simulink model "CACC_system_struct"  (Simulink 8.2)
settings: Solver=ode1  SolverMode=SingleTasking  StartTime=0.0  StopTime=inf  FixedStep=0.01  RelTol=1e-3
PreLoadFcn:
  | numd_dvsp = [0.3579 0 -0.3579];
  | dend_dvsp = [1 -1.846 0.8535];
  | simpleacc_param
PostLoadFcn:
  | , if any(exist('dsrtsu_mdlpostloadfcn', 'file') == [2, 3, 6]), try dsrtsu_mdlpostloadfcn('Execute', bdroot); catch fprintf('Error in PostLoadFcn (dsrtsu_mdlpostloadfcn) for model "%s":\n %s\n', bdroot, lasterr); end, end,
undefined symbols (not defined in the file or in its folder): command_mode, max_accel_m_s2, override_enabled, speed_command_m_s, wrench_effort_command
libraries: carma_platform x3, dsrc_transmitter x2, rtitttasklib x2, lightbar x2, srx_platform x1
(part 4 of 4)

== matlab function CACC Control Code 1/Coordination/MATLAB Function ==
  data: u input double; y output double
function y = fcn(u)
%#codegen

y=veh_pos(u);


function y_out=veh_pos(x)

%N=length(x);
cacc_grp_len=x(16);

z=zeros(1,15);
        if (cacc_grp_len == 2)                %% always put the subject vehicle at Virtual Position 1 in the Vector Forming            
                A=[x(2); x(5)];
                b=[x(3); x(6)];            
        elseif (cacc_grp_len == 3)            
                A=[x(2); x(5); x(8)];
                b=[x(3); x(6); x(9)];             
        elseif (cacc_grp_len == 4)           
                A=[x(2); x(5); x(8); x(11)];
                b=[x(3); x(6); x(9); x(12)];          
        elseif (cacc_grp_len == 5)            
                A=[x(2); x(5); x(8); x(11); x(14)];
                b=[x(3); x(6); x(9); x(12); x(15)];            
        else
             A=[x(2)];
             b=[x(3)];
        end
    
    a=A\b;
 
    alpha=atan(a(1));    %% angle of moving axle w.r.t. to East of the original coordinate system
    
    alpha=pi/2.0-alpha;  %% angle of moving axle w.r.t. to North of the original coordinate system
    alpha=-alpha;        %% so that the original y-axis is in the Miving Axle direction;
    
    
    if (cacc_grp_len == 2)                %% always put the subject vehicle at Virtual Position 1 in the Vector Forming         
            p1_2=Coord_Trans(alpha,A(1),b(1),A(2),b(2));
            tmp=[0 p1_2(2)];
            [Ord, Ind]=sort(tmp, 'descend');
            
            z(1)=x(1); %%BSM1: ID
            z(2)=Ind(1); %%BSM1: Contol Pos
            z(3)=0; %%BSM1: Lane ID
            z(4)=x(4); %%BSM2: ID
            z(5)=Ind(2); %%BSM2: Contol Pos
            z(6)=0; %%BSM2: Lane ID
            z(7)=-1; %%BSM3: ID
            z(8)=-1; %%BSM3: Contol Pos
            z(9)=-1; %%BSM3: Lane ID
            z(10)=-1; %%BSM4: ID
            z(11)=-1; %%BSM4: Contol Pos
            z(12)=-1; %%BSM4: Lane ID
            z(13)=-1; %%BSM5: ID
            z(14)=-1; %%BSM5: Contol Pos
            z(15)=-1; %%BSM5: Lane ID

            
   elseif (cacc_grp_len == 3)
            p1_2=Coord_Trans(alpha,A(1),b(1),A(2),b(2));
            p1_3=Coord_Trans(alpha,A(1),b(1),A(3),b(3));
            tmp=[0 p1_2(2) p1_3(2)];
            [Ord, Ind]=sort(tmp, 'descend');
            
            z(1)=x(1); %%BSM1: ID
            z(2)=Ind(1); %%BSM1: Contol Pos
            z(3)=0; %%BSM1: Lane ID
            z(4)=x(4); %%BSM2: ID
            z(5)=Ind(2); %%BSM2: Contol Pos
            z(6)=0; %%BSM2: Lane ID
            z(7)=x(7); %%BSM3: ID
            z(8)=Ind(3); %%BSM3: Contol Pos
            z(9)=0; %%BSM3: Lane ID
            z(10)=-1; %%BSM4: ID
            z(11)=-1; %%BSM4: Contol Pos
            z(12)=-1; %%BSM4: Lane ID
            z(13)=-1; %%BSM5: ID
            z(14)=-1; %%BSM5: Contol Pos
            z(15)=-1; %%BSM5: Lane ID
                     
    elseif (cacc_grp_len == 4)
            p1_2=Coord_Trans(alpha,A(1),b(1),A(2),b(2));
            p1_3=Coord_Trans(alpha,A(1),b(1),A(3),b(3));
            p1_4=Coord_Trans(alpha,A(1),b(1),A(4),b(4));
            tmp=[0 p1_2(2) p1_3(2) p1_4(2)];
            [Ord, Ind]=sort(tmp, 'descend');
            
            z(1)=x(1); %%BSM1: ID
            z(2)=Ind(1); %%BSM1: Contol Pos
            z(3)=0; %%BSM1: Lane ID
            z(4)=x(4); %%BSM2: ID
            z(5)=Ind(2); %%BSM2: Contol Pos
            z(6)=0; %%BSM2: Lane ID
            z(7)=x(7); %%BSM3: ID
            z(8)=Ind(3); %%BSM3: Contol Pos
            z(9)=0; %%BSM3: Lane ID
            z(10)=x(10); %%BSM4: ID
            z(11)=Ind(4); %%BSM4: Contol Pos
            z(12)=0; %%BSM4: Lane ID
            z(13)=-1; %%BSM5: ID
            z(14)=-1; %%BSM5: Contol Pos
            z(15)=-1; %%BSM5: Lane ID
                
    elseif (cacc_grp_len == 5)
            p1_2=Coord_Trans(alpha,A(1),b(1),A(2),b(2));
            p1_3=Coord_Trans(alpha,A(1),b(1),A(3),b(3));
            p1_4=Coord_Trans(alpha,A(1),b(1),A(4),b(4));         
            p1_5=Coord_Trans(alpha,A(1),b(1),A(5),b(5));
            tmp=[0 p1_2(2) p1_3(2) p1_4(2) p1_5(2)];            
            [Ord, Ind]=sort(tmp, 'descend');
            
            z(1)=x(1);  
            z(2)=Ind(1); %%BSM1: Contol Pos
            z(3)=0; %%BSM1: Lane ID
            z(4)=x(4); %%BSM2: ID
            z(5)=Ind(2); %%BSM2: Contol Pos
            z(6)=0; %%BSM2: Lane ID
            z(7)=x(7); %%BSM3: ID
            z(8)=Ind(3); %%BSM3: Contol Pos
            z(9)=0; %%BSM3: Lane ID
            z(10)=x(10); %%BSM4: ID
            z(11)=Ind(4); %%BSM4: Contol Pos
            z(12)=0; %%BSM4: Lane ID
            z(13)=x(13); %%BSM5: ID
            z(14)=Ind(5); %%BSM5: Contol Pos
            z(15)=0; %%BSM5: Lane ID
    else           
            z(1)=x(1); %%BSM1: ID
            z(2)=1; %%BSM1: Contol Pos
            z(3)=0; %%BSM1: Lane ID
            z(4)=-1; %%BSM2: ID
            z(5)=-1; %%BSM2: Contol Pos
            z(6)=-1; %%BSM2: Lane ID
            z(7)=-1; %%BSM3: ID
            z(8)=-1; %%BSM3: Contol Pos
            z(9)=-1; %%BSM3: Lane ID
            z(10)=-1; %%BSM4: ID
            z(11)=-1; %%BSM4: Contol Pos
            z(12)=-1; %%BSM4: Lane ID
            z(13)=-1; %%BSM5: ID
            z(14)=-1; %%BSM5: Contol Pos
            z(15)=-1; %%BSM5: Lane ID
    end
    y_out=z;

%end


function local  = Coord_Trans(alpha, subj_x, subj_y, x, y)

    alpha=pi/2.0-alpha;  %% angle of moving axle w.r.t. to North of the original coordinate system
    alpha=-alpha;        %% so that the original y-axis is in the Miving Axle direction;
    
    R=[cos(alpha) sin(alpha); -sin(alpha) cos(alpha)];
    
    p1=[subj_x; subj_y];  %% coordinate of p1 in old system
    p2=[x;y];  %% coordinate of p2 in old system
  
  local = R*(p2-p1);   
%end
